simulink model "Green_Ball_Tracking_Mounted"  (R2016a)
settings: configuration reference "AR_Drone_ConfigSet" (kept outside this file)
undefined symbols (not defined in the file): Drone_StateModeType, sigbuilder_block
libraries: simulink x10, AR_Drone_Sensors x2, AR_Drone_Actuators x2, AR_Drone_Video x1, AR_Drone_Positioning x1
(part 1 of 2)
settings Model: DataDictionary=ArDroneDataDictionary.sldd  SimulationMode=external  ExtModeTrigDuration=48000  Creator=nraman  LastModifiedBy=sannem
settings ConfigSetRef: Description='192.168.1.1' 1 17725  DDName=ArDroneDataDictionary.sldd

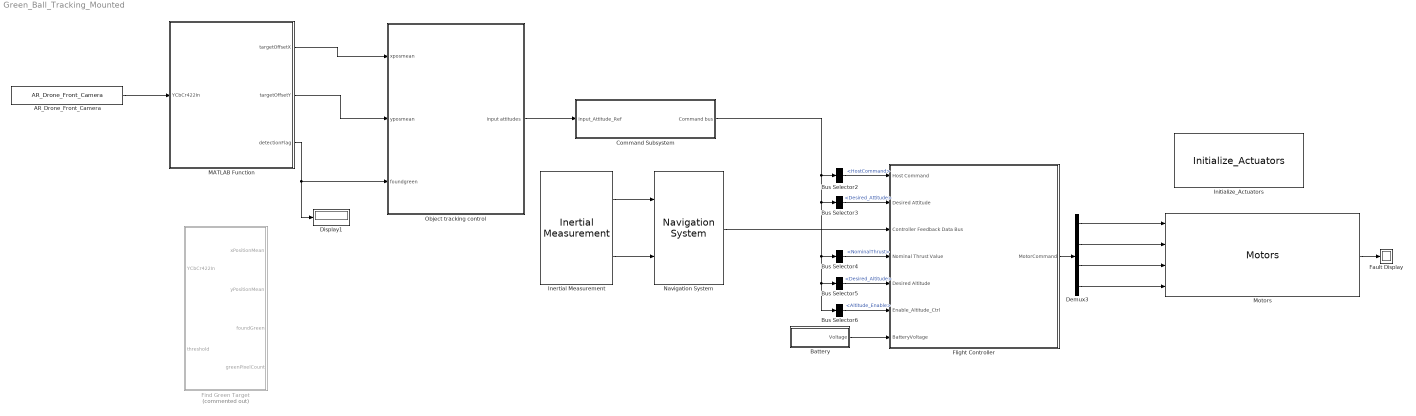
== system Green_Ball_Tracking_Mounted ==
  AR_Drone_Front_Camera : AR_Drone_Video/AR_Drone_Front_Camera  SFunctionSpec=videoGrabImage1(uint8 y1[1843200])  SampleTime=0.1  ShowSpec=off
  Battery : Subsystem
  Bus Selector2 : BusSelector  OutputSignals=HostCommand
  Bus Selector3 : BusSelector  OutputSignals=Desired_Attitude
  Bus Selector4 : BusSelector  OutputSignals=NominalThrust
  Bus Selector5 : BusSelector  OutputSignals=Desired_Altitude
  Bus Selector6 : BusSelector  OutputSignals=Altitude_Enable
  Command Subsystem : Subsystem
  Demux3 : Demux
  Display1 : Display
  Fault Display : Display
  Find Green Target : MATLAB Function  Commented=on  TreatAsAtomicUnit=on  mask(Average Green Position){width=1280, height=720, downScaleFactor=5}
      mask prompts: width "Horizontal resolution"; height "Vertical resolution"; downScaleFactor "Video downscale factor"
      mask help: This block returns the average x and y coordinates of all green pixels within the YCbCr 4:2:2 format input video. Specifying the downscaling factor results in the input video being downsampled by that factor in both horizontal and vertical direction to reduce computation time. The input threshold [0 - 255] controls how "green" high the red and blue shift of the pixels must be before they are no longer considered green.
  Flight Controller : Subsystem
  Inertial Measurement : AR_Drone_Sensors/Inertial Measurement  Ts=1/400
  Initialize_Actuators : AR_Drone_Actuators/Initialize_Actuators  ShowSpec=on
  MATLAB Function : MATLAB Function  TreatAsAtomicUnit=on  mask(AR Drone:  Find Colored Object Position){width=1280, height=720, downScaleFactor=5, cbFloor=0, cbCeiling=117, crFloor=0, crCeiling=117, pixelThreshold=10}
      mask prompts: width "Video input width"; height "Video input height"; downScaleFactor "Video down sample factor"; cbFloor "Blue shift minimum [0-255]"; cbCeiling "Blue shift maximum [0-255]"; crFloor "Red shift minimum [0-255]"; crCeiling "Red shift maximum [0-255]"; pixelThreshold "Minimum object detection pixel count"
      mask help:
      | This MATLAB function block takes an input video stream, down samples in both the horizontal and veritcal direction to reduce the computational demand, and then determines how many pixels fall within the user specified colorspace region and what their average postition is in the video. If you are experiencing some artifacts which are hard to tune out, increase the minimum target pixel count. No target will be registered (detectionFlag = 0) unless as many pixels as you define are found in the target colorspace (detectionFlag = 1).
      | The output x and y position are scaled between -1 and 1.
      |
      | Using the YCbCr colorspace some recommend values are:
      |
      | Green target:
      | cb[min, max] = [0, 100]
      | cr[min, max] = [0, 100]
      |
      | Blue target:
      | cb[min, max] = [155, 255]
      | cr[min, max] = [0, 100]
      |
      | Red target:
      | cb[min, max] = [0, 100]
      | cr[min, max] = [155, 255]
  Motors : AR_Drone_Actuators/Motors
  Navigation System : AR_Drone_Positioning/Navigation System
  Object tracking control : Subsystem  mask{HorRes=1280, VerRes=720}
      mask prompts: HorRes "Horizontal resolution"; VerRes "VerticalResolution"
  wires:
  Motors/1 -> Fault Display/1
  Demux3/1 -> Motors/1
  Demux3/2 -> Motors/2
  Demux3/3 -> Motors/3
  Demux3/4 -> Motors/4
  Inertial Measurement/1 -> Navigation System/1
  Inertial Measurement/2 -> Navigation System/2
  Command Subsystem/1(Command bus) -> Bus Selector2/1, Bus Selector3/1, Bus Selector6/1, Bus Selector5/1, Bus Selector4/1
  Bus Selector4/1 -> Flight Controller/4(Nominal Thrust Value)  "<NominalThrust>"
  Bus Selector5/1 -> Flight Controller/5(Desired Altitude)  "<Desired_Altitude>"
  Bus Selector6/1 -> Flight Controller/6(Enable_Altitude_Ctrl)  "<Altitude_Enable>"
  Flight Controller/1(MotorCommand) -> Demux3/1
  Bus Selector2/1 -> Flight Controller/1(Host Command)  "<HostCommand>"
  Bus Selector3/1 -> Flight Controller/2(Desired Attitude)  "<Desired_Attitude>"
  Navigation System/1 -> Flight Controller/3(Controller Feedback Data Bus)
  AR_Drone_Front_Camera/1 -> MATLAB Function/1(YCbCr422In)
  Object tracking control/1(input attitudes) -> Command Subsystem/1(Input_Attitude_Ref)
  Battery/1(Voltage) -> Flight Controller/7(BatteryVoltage)
  MATLAB Function/1(targetOffsetX) -> Object tracking control/1(xposmean)
  MATLAB Function/2(targetOffsetY) -> Object tracking control/2(yposmean)
  MATLAB Function/3(detectionFlag) -> Display1/1, Object tracking control/3(foundgreen)

== system Green_Ball_Tracking_Mounted/Battery ==
  Battery Voltage Measurement : AR_Drone_Sensors/Battery Voltage Measurement  SFunctionSpec=void BatteryMeasure_step(single y1[1])  SampleTime=-1
  Deci-Volts to Volts : Gain  Gain=1/10
  Display6 : Display
  Voltage : Outport
  wires:
  Deci-Volts to Volts/1 -> Voltage/1, Display6/1
  Battery Voltage Measurement/1 -> Deci-Volts to Volts/1

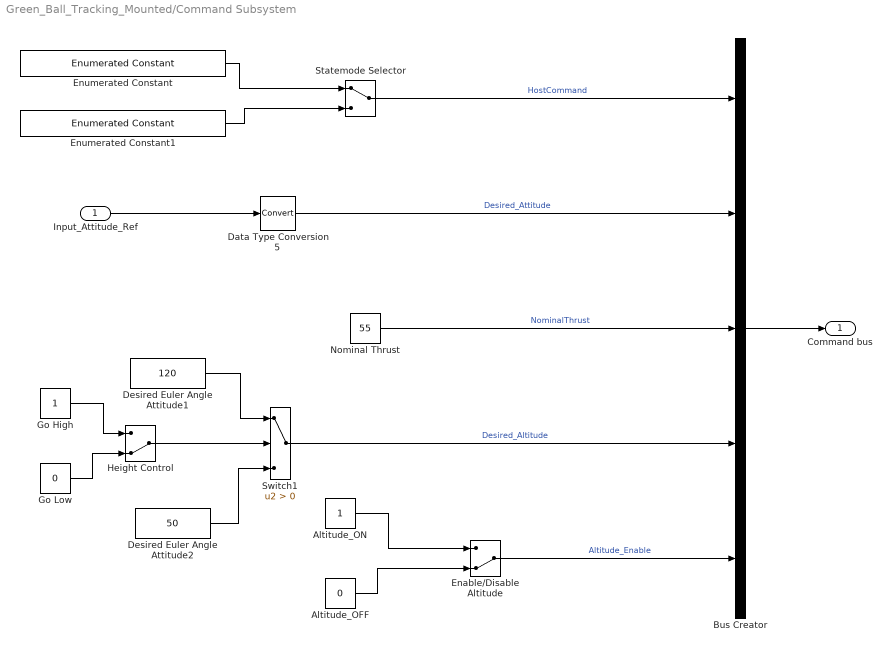
== system Green_Ball_Tracking_Mounted/Command Subsystem ==
  Input_Attitude_Ref : Inport
  Altitude_OFF : Constant  Value=0
  Altitude_ON : Constant
  Bus Creator : BusCreator  Inputs=5
  Data Type Conversion5 : DataTypeConversion
  Desired Euler Angle Attitude1 : Constant  Value=120
  Desired Euler Angle Attitude2 : Constant  Value=50
  Enable/Disable Altitude : ManualSwitch  CurrentSetting=0
  Enumerated Constant : simulink/Sources/Enumerated Constant  OutDataTypeStr=Enum: Drone_StateModeType  Value=Drone_StateModeType.Controlled_Flight  SampleTime=inf
      settings: AttributesFormatString=%<Value>
  Enumerated Constant1 : simulink/Sources/Enumerated Constant  OutDataTypeStr=Enum: Drone_StateModeType  Value=Drone_StateModeType.Landing_Sequence  SampleTime=inf
      settings: AttributesFormatString=%<Value>
  Go High : Constant
  Go Low : Constant  Value=0
  Height Control : ManualSwitch  CurrentSetting=0
  Nominal Thrust : Constant  Value=55
  "Statemode Selector " : ManualSwitch
  Switch1 : Switch  Criteria=u2 > Threshold
  Command bus : Outport
  wires:
  Desired Euler Angle Attitude2/1 -> Switch1/3
  Height Control/1 -> Switch1/2
  Desired Euler Angle Attitude1/1 -> Switch1/1
  Go High/1 -> Height Control/1
  Go Low/1 -> Height Control/2
  Altitude_OFF/1 -> Enable/Disable Altitude/2
  Altitude_ON/1 -> Enable/Disable Altitude/1
  Switch1/1 -> Bus Creator/4  "Desired_Altitude"
  Enable/Disable Altitude/1 -> Bus Creator/5  "Altitude_Enable"
  Nominal Thrust/1 -> Bus Creator/3  "NominalThrust"
  Input_Attitude_Ref/1 -> Data Type Conversion5/1
  Data Type Conversion5/1 -> Bus Creator/2  "Desired_Attitude"
  "Statemode Selector "/1 -> Bus Creator/1  "HostCommand"
  Enumerated Constant/1 -> "Statemode Selector "/1
  Enumerated Constant1/1 -> "Statemode Selector "/2
  Bus Creator/1 -> Command bus/1

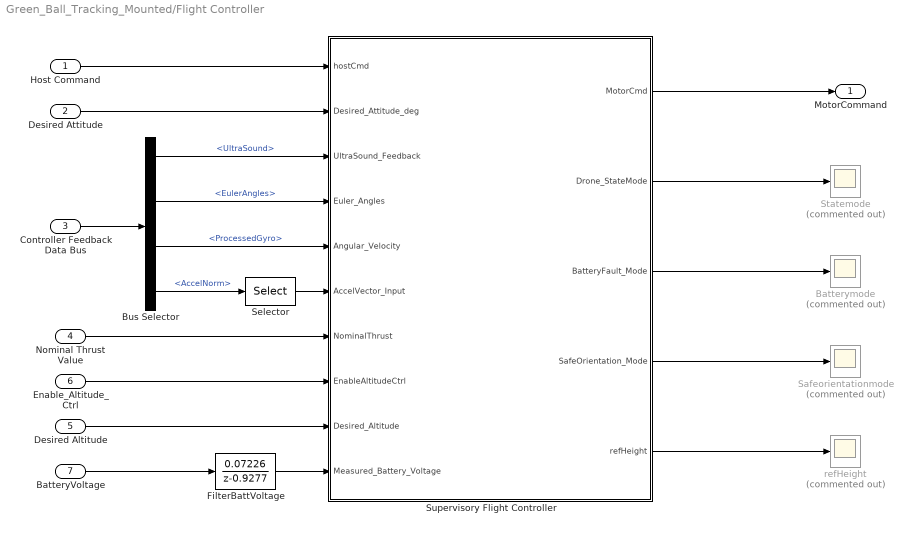
== system Green_Ball_Tracking_Mounted/Flight Controller ==
  Host Command : Inport
  Desired Attitude : Inport  Port=2
  Controller Feedback Data Bus : Inport  Port=3
  Nominal Thrust Value : Inport  Port=4
  Desired Altitude : Inport  Port=5
  Enable_Altitude_Ctrl : Inport  Port=6
  BatteryVoltage : Inport  Port=7
  Batterymode : Scope  Commented=on
  Bus Selector : BusSelector  OutputSignals=UltraSound,EulerAngles,ProcessedGyro,AccelNorm
  FilterBattVoltage : DiscreteTransferFcn  Numerator=[ 0.07226]  Denominator=[1 -0.9277]
  Safeorientationmode : Scope  Commented=on
  Selector : Selector  InputPortWidth=3  IndexOptions=Index vector (dialog)  Indices=[3]  OutputSizes=1
  Statemode : Scope  Commented=on
  Supervisory Flight Controller : Stateflow chart  TreatAsAtomicUnit=on
  refHeight : Scope  Commented=on
  MotorCommand : Outport
  wires:
  Supervisory Flight Controller/1(MotorCmd) -> MotorCommand/1
  Desired Attitude/1 -> Supervisory Flight Controller/2(Desired_Attitude_deg)
  Desired Altitude/1 -> Supervisory Flight Controller/9(Desired_Altitude)
  Supervisory Flight Controller/2(" Drone_StateMode") -> Statemode/1
  Host Command/1 -> Supervisory Flight Controller/1(hostCmd)
  Bus Selector/1 -> Supervisory Flight Controller/3(UltraSound_Feedback)  "<UltraSound>"
  Nominal Thrust Value/1 -> Supervisory Flight Controller/7(NominalThrust)
  Controller Feedback Data Bus/1 -> Bus Selector/1
  Enable_Altitude_Ctrl/1 -> Supervisory Flight Controller/8(EnableAltitudeCtrl)
  BatteryVoltage/1 -> FilterBattVoltage/1
  FilterBattVoltage/1 -> Supervisory Flight Controller/10(Measured_Battery_Voltage)
  Selector/1 -> Supervisory Flight Controller/6(AccelVector_Input)
  Bus Selector/4 -> Selector/1  "<AccelNorm>"
  Bus Selector/2 -> Supervisory Flight Controller/4(Euler_Angles)  "<EulerAngles>"
  Bus Selector/3 -> Supervisory Flight Controller/5(Angular_Velocity)  "<ProcessedGyro>"
  Supervisory Flight Controller/3(" BatteryFault_Mode") -> Batterymode/1
  Supervisory Flight Controller/4(" SafeOrientation_Mode") -> Safeorientationmode/1
  Supervisory Flight Controller/5(refHeight) -> refHeight/1

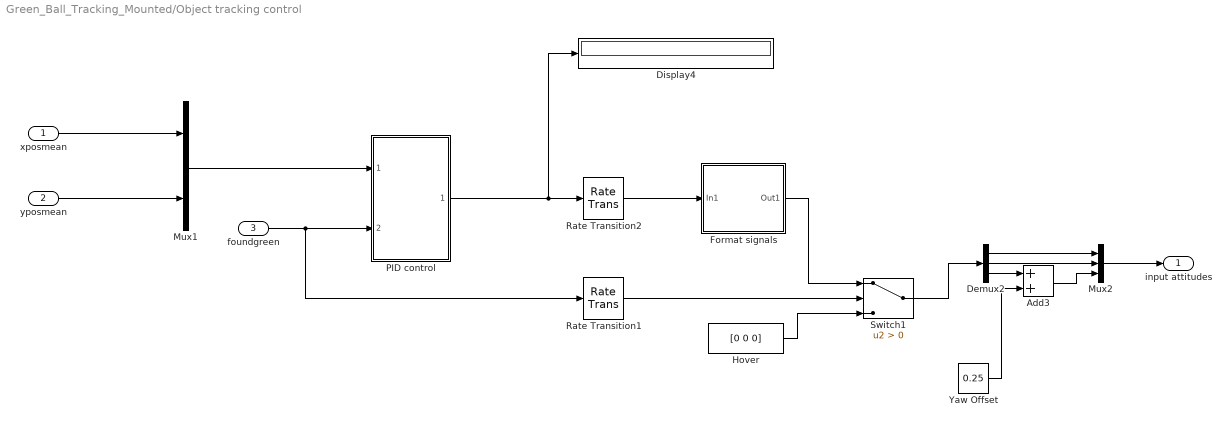
== system Green_Ball_Tracking_Mounted/Object tracking control ==
  xposmean : Inport
  yposmean : Inport  Port=2
  foundgreen : Inport  Port=3
  Add3 : Sum
  Demux2 : Demux  Outputs=3
  Display4 : Display
  Format signals : Subsystem
  Hover : Constant  Value=[0 0 0]
  Mux1 : Mux  Inputs=2
  Mux2 : Mux  Inputs=3
  PID control : Subsystem
  Rate Transition1 : RateTransition
  Rate Transition2 : RateTransition
  Switch1 : Switch  Criteria=u2 > Threshold
  "Yaw Offset " : Constant  Value=0.25
  input attitudes : Outport
  wires:
  Switch1/1 -> Demux2/1
  "Yaw Offset "/1 -> Add3/2
  Demux2/2 -> Mux2/2
  Demux2/1 -> Mux2/1
  Demux2/3 -> Add3/1
  Mux2/1 -> input attitudes/1
  Add3/1 -> Mux2/3
  foundgreen/1 -> PID control/2(Reset Trigger), Rate Transition1/1
  Rate Transition1/1 -> Switch1/2
  Hover/1 -> Switch1/3
  xposmean/1 -> Mux1/1
  yposmean/1 -> Mux1/2
  Rate Transition2/1 -> Format signals/1(In1)
  Format signals/1(Out1) -> Switch1/1
  PID control/1(Control output) -> Display4/1, Rate Transition2/1
  Mux1/1 -> PID control/1(XY Input)

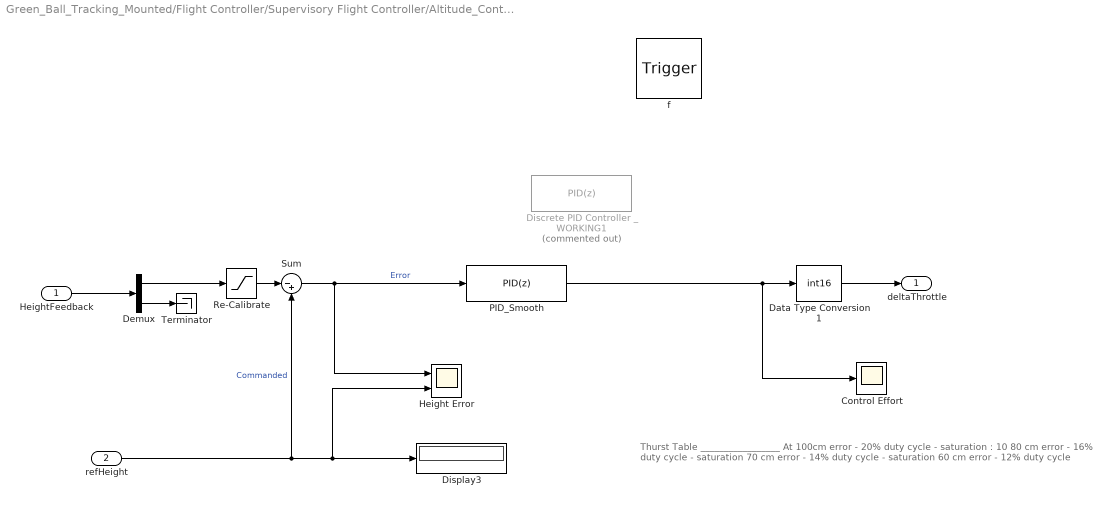
== system Green_Ball_Tracking_Mounted/Flight Controller/Supervisory Flight Controller/Altitude_Control ==
  note: Thurst Table
      | _________________
      | At 100cm error  - 20% duty cycle - saturation : 10
      | 80 cm error - 16% duty cycle - saturation
      | 70 cm error - 14% duty cycle - saturation
      | 60 cm error - 12% duty cycle
  HeightFeedback : Inport  OutDataTypeStr=double  PortDimensions=2
  refHeight : Inport  Port=2  OutDataTypeStr=double  PortDimensions=1
  f : TriggerPort  TriggerType=function-call  VariantControl=Variant
      settings: CopyFcn=Stateflow.SLINSF.SimulinkMan.removeBlockPreDeleteFcn  PreDeleteFcn=Stateflow.SLINSF.SimulinkMan.unsafePredeleteFcn
  Control Effort : Scope
  Data Type Conversion1 : DataTypeConversion  OutDataTypeStr=int16
  Demux : Demux  Outputs=2
  Discrete PID Controller _ WORKING1 : simulink/Continuous/PID Controller  Commented=on  Controller=PID  TimeDomain=Discrete-time  SampleTime=-1  IntegratorMethod=Forward Euler  FilterMethod=Forward Euler  Form=Parallel  UseFilter=on  ControllerParametersSource=internal  P=0.387369235850492*0.7  I=0.018136*4  D=0.819231727791919*0.15  N=12.5907330811849  InitialConditionSource=internal  InitialConditionForIntegrator=0  InitialConditionForFilter=0  ExternalReset=none  LimitOutput=on  UpperSaturationLimit=20  LowerSaturationLimit=-20  LinearizeAsGain=off  AntiWindupMode=clamping  Kb=1  TrackingMode=off  Kt=1  PParamMin=[]  PParamMax=[]  IParamMin=[]  IParamMax=[]  DParamMin=[]  DParamMax=[]  NParamMin=[]  NParamMax=[]  KbParamMin=[]  KbParamMax=[]  KtParamMin=[]  KtParamMax=[]  POutMin=[]  POutMax=[]  IOutMin=[]  IOutMax=[]  DOutMin=[]  DOutMax=[]  NOutMin=[]  NOutMax=[]  KbOutMin=[]  KbOutMax=[]  KtOutMin=[]  KtOutMax=[]  IntegratorOutMin=[]  IntegratorOutMax=[]  FilterOutMin=[]  FilterOutMax=[]  SumOutMin=[]  SumOutMax=[]  SumI1OutMin=[]  SumI1OutMax=[]  SumI2OutMin=[]  SumI2OutMax=[]  SumI3OutMin=[]  SumI3OutMax=[]  SumDOutMin=[]  SumDOutMax=[]  SaturationOutMin=[]  SaturationOutMax=[]  IntegratorContinuousStateAttributes=''  IntegratorStateMustResolveToSignalObject=off  IntegratorRTWStateStorageClass=Auto  FilterContinuousStateAttributes=''  FilterStateMustResolveToSignalObject=off  FilterRTWStateStorageClass=Auto  DifferentiatorICPrevScaledInput=0  DifferentiatorOutMin=[]  DifferentiatorOutMax=[]
  Display3 : Display
  Height Error : Scope  NumInputPorts=2
  PID_Smooth : simulink/Continuous/PID Controller  Controller=PID  TimeDomain=Discrete-time  SampleTime=-1  IntegratorMethod=Forward Euler  FilterMethod=Forward Euler  Form=Parallel  UseFilter=on  ControllerParametersSource=internal  P=0.387369235850492*0.9  I=0.018136*4  D=0.819231727791919*0.2  N=12.5907330811849  InitialConditionSource=internal  InitialConditionForIntegrator=0  InitialConditionForFilter=0  ExternalReset=none  LimitOutput=on  UpperSaturationLimit=20  LowerSaturationLimit=-20  LinearizeAsGain=off  AntiWindupMode=clamping  Kb=1  TrackingMode=off  Kt=1  PParamMin=[]  PParamMax=[]  IParamMin=[]  IParamMax=[]  DParamMin=[]  DParamMax=[]  NParamMin=[]  NParamMax=[]  KbParamMin=[]  KbParamMax=[]  KtParamMin=[]  KtParamMax=[]  POutMin=[]  POutMax=[]  IOutMin=[]  IOutMax=[]  DOutMin=[]  DOutMax=[]  NOutMin=[]  NOutMax=[]  KbOutMin=[]  KbOutMax=[]  KtOutMin=[]  KtOutMax=[]  IntegratorOutMin=[]  IntegratorOutMax=[]  FilterOutMin=[]  FilterOutMax=[]  SumOutMin=[]  SumOutMax=[]  SumI1OutMin=[]  SumI1OutMax=[]  SumI2OutMin=[]  SumI2OutMax=[]  SumI3OutMin=[]  SumI3OutMax=[]  SumDOutMin=[]  SumDOutMax=[]  SaturationOutMin=[]  SaturationOutMax=[]  IntegratorContinuousStateAttributes=''  IntegratorStateMustResolveToSignalObject=off  IntegratorRTWStateStorageClass=Auto  FilterContinuousStateAttributes=''  FilterStateMustResolveToSignalObject=off  FilterRTWStateStorageClass=Auto  DifferentiatorICPrevScaledInput=0  DifferentiatorOutMin=[]  DifferentiatorOutMax=[]
  Re-Calibrate : Saturate  UpperLimit=200  LowerLimit=0  OutMin=0  OutMax=200
      settings: AttributesFormatString=|
      | Upper: %<UpperLimit>
      | Lower %<LowerLimit>
  Sum : Sum  Inputs=|-+
  Terminator : Terminator
  deltaThrottle : Outport  OutDataTypeStr=int16
  wires:
  refHeight/1 -> Sum/2, Height Error/2, Display3/1  "Commanded"
  PID_Smooth/1 -> Control Effort/1, Data Type Conversion1/1
  Data Type Conversion1/1 -> deltaThrottle/1
  HeightFeedback/1 -> Demux/1
  Demux/1 -> Re-Calibrate/1
  Sum/1 -> PID_Smooth/1, Height Error/1  "Error"
  Re-Calibrate/1 -> Sum/1
  Demux/2 -> Terminator/1

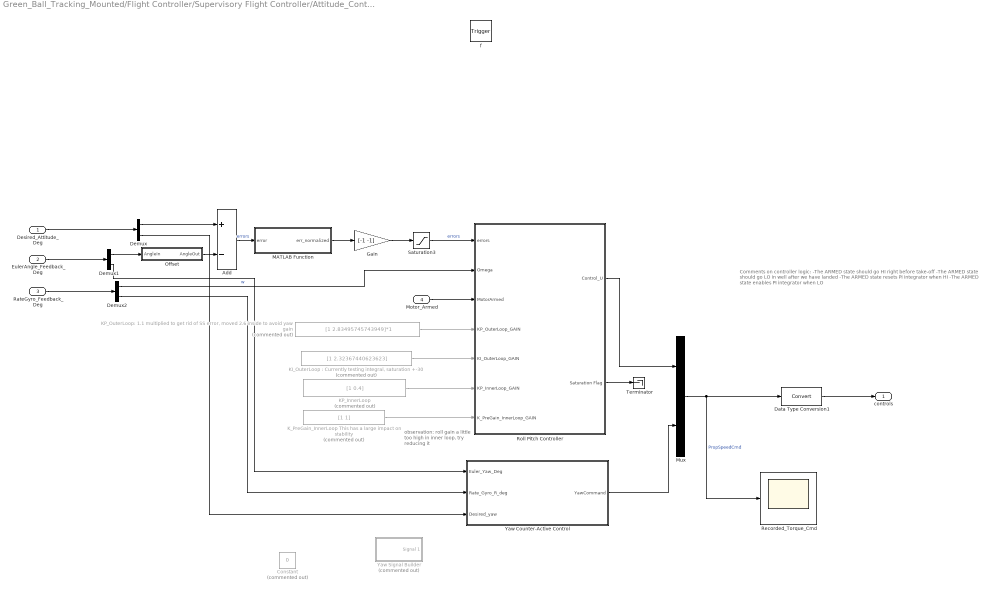
== system Green_Ball_Tracking_Mounted/Flight Controller/Supervisory Flight Controller/Attitude_Control ==
  note: observation:
      | roll gain a little
      | too high in inner
      | loop, try reducing it
  note: Comments on controller logic:
      | -The ARMED state should go HI right before take-off
      | -The  ARMED state should go LO in well after we have landed
      | -The ARMED state resets PI integrator when HI
      | -The ARMED state enables PI integrator when LO
  Desired_Attitude_Deg : Inport  OutDataTypeStr=double  PortDimensions=3
  EulerAngle_Feedback_Deg : Inport  Port=2  OutDataTypeStr=double  PortDimensions=3
  RateGyro_Feedback_Deg : Inport  Port=3  OutDataTypeStr=double  PortDimensions=3
  Motor_Armed : Inport  Port=4  OutDataTypeStr=double  PortDimensions=1
  f : TriggerPort  TriggerType=function-call  VariantControl=Variant
      settings: CopyFcn=Stateflow.SLINSF.SimulinkMan.removeBlockPreDeleteFcn  PreDeleteFcn=Stateflow.SLINSF.SimulinkMan.unsafePredeleteFcn
  Add : Sum  Inputs=+-  AccumDataTypeStr=single  OutDataTypeStr=single
  Constant : Constant  Commented=on  Value=0
  Data Type Conversion1 : DataTypeConversion
  Demux : Demux  Outputs=[2 1]
  Demux1 : Demux  Outputs=[2 1]
  Demux2 : Demux  Outputs=[2 1]
  Gain : Gain  Gain=[-1 -1]
  "KI_OuterLoop : Currently testing integral, saturation +-30" : Constant  Commented=on  Value=[1 2.32367440623623]
  KP_InnerLoop : Constant  Commented=on  Value=[1 0.4]
  "KP_OuterLoop: 1.1 multiplied to get rid of SS error, moved 2.6 inside to avoid yaw gain" : Constant  Commented=on  Value=[1 2.83495745743949]*1
  K_PreGain_InnerLoop This has a large impact on stability : Constant  Commented=on  Value=[1 1]
  MATLAB Function : MATLAB Function  TreatAsAtomicUnit=on
  Mux : Mux  Inputs=2
  Offset : Subsystem
  Recorded_Torque_Cmd : Scope
  Roll Pitch Controller : Subsystem  TreatAsAtomicUnit=on
  Saturation3 : Saturate  UpperLimit=[25 25]  LowerLimit=[-25 -25]  OutDataTypeStr=single
      settings: AttributesFormatString=%<LowerLimit> to %<UpperLimit>
  Terminator : Terminator
  Yaw Counter-Active Control : Subsystem
  "Yaw Signal Builder " : Subsystem  Tag=STV Subsys  Commented=on  LoadFcn=sigbuilder_block('load');  StartFcn=sigbuilder_block('start');  StopFcn=sigbuilder_block('stop');  ClipboardFcn=sigbuilder_block('clipboard');  mask(Sigbuilder block){}
      mask help: Simulink:masks:SigbuilderBlock_MD
      mask init:
      | if ~strcmp(get_param(bdroot(gcbh),'SimulationStatus'),'stopped') tuvar = sigbuilder_block('maskInit'); end
      settings: CopyFcn=sigbuilder_block('copy');  DeleteFcn=sigbuilder_block('delete');  ModelCloseFcn=sigbuilder_block('modelClose');  PreSaveFcn=sigbuilder_block('preSave');  PauseFcn=sigbuilder_block('pause');  ContinueFcn=sigbuilder_block('continue');  NameChangeFcn=sigbuilder_block('namechange');  OpenFcn=sigbuilder_block('open',[437.25 118.5 550.5 394.5 ]);  CloseFcn=sigbuilder_block('close');
      mask Display: plot(0, 0, 100, 100,[2, 2, 32, 32, 2], [68, 8, 8, 68, 68],[32, 2], [38, 38], [32, 19, 2],[53, 60, 44], [32, 17, 17, 2],[16, 16, 31, 31]);txt = getActiveGroup(gcbh);text(2, 100, txt,'verticalAlignment', 'top');
  controls : Outport  OutDataTypeStr=int16  PortDimensions=3  InitialOutput=0
  wires:
  Add/1 -> MATLAB Function/1(error)  "errors"
  Demux1/1 -> Offset/1(AngleIn)
  Demux2/1 -> Roll Pitch Controller/2(Omega)  "w"
  KP_InnerLoop/1 -> Roll Pitch Controller/6(KP_InnerLoop_GAIN)
  "KP_OuterLoop: 1.1 multiplied to get rid of SS error, moved 2.6 inside to avoid yaw gain"/1 -> Roll Pitch Controller/4(KP_OuterLoop_GAIN)
  K_PreGain_InnerLoop This has a large impact on stability/1 -> Roll Pitch Controller/7(K_PreGain_InnerLoop_GAIN)
  "KI_OuterLoop : Currently testing integral, saturation +-30"/1 -> Roll Pitch Controller/5(KI_OuterLoop_GAIN)
  Saturation3/1 -> Roll Pitch Controller/1(errors)  "errors"
  MATLAB Function/1(err_normalized) -> Gain/1
  Gain/1 -> Saturation3/1
  Roll Pitch Controller/2(Saturation Flag) -> Terminator/1
  Demux/1 -> Add/1
  Roll Pitch Controller/1(Control_U) -> Mux/1
  Offset/1(AngleOut) -> Add/2
  Demux2/2 -> Yaw Counter-Active Control/2(Rate_Gyro_R_deg)
  Yaw Counter-Active Control/1(YawCommand) -> Mux/2
  Desired_Attitude_Deg/1 -> Demux/1
  EulerAngle_Feedback_Deg/1 -> Demux1/1
  RateGyro_Feedback_Deg/1 -> Demux2/1
  Motor_Armed/1 -> Roll Pitch Controller/3(MotorArmed)
  Demux1/2 -> Yaw Counter-Active Control/1(Euler_Yaw_Deg)
  Data Type Conversion1/1 -> controls/1
  Mux/1 -> Data Type Conversion1/1, Recorded_Torque_Cmd/1  "PropSpeedCmd"
  Demux/2 -> Yaw Counter-Active Control/3("Desired_yaw ")

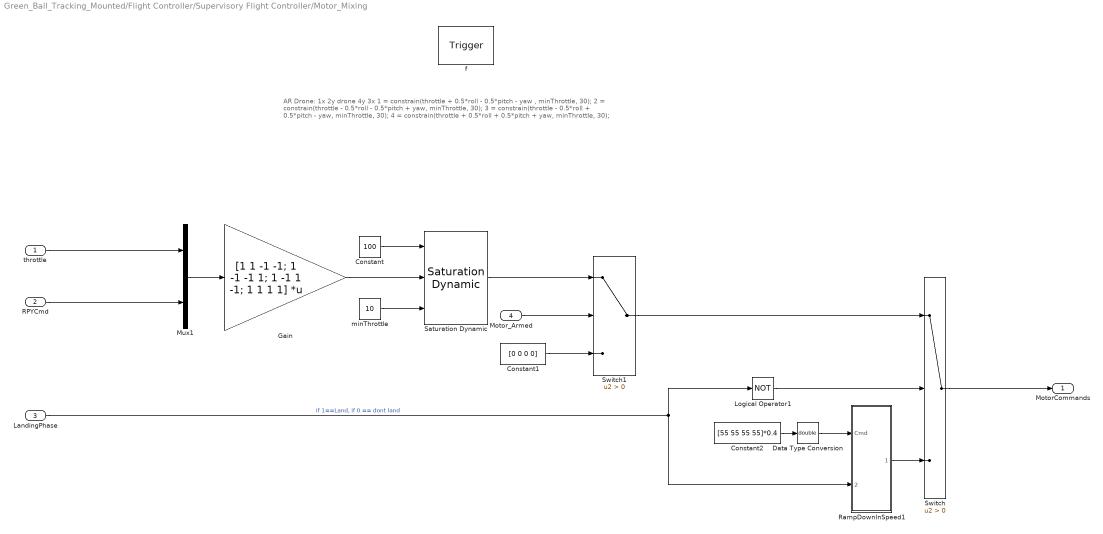
== system Green_Ball_Tracking_Mounted/Flight Controller/Supervisory Flight Controller/Motor_Mixing ==
  note: AR Drone:
      |
      |   1x         2y
      |      drone
      |   4y         3x
      |
      |  1 = constrain(throttle + 0.5*roll - 0.5*pitch - yaw , minThrottle, 30);
      |  2 = constrain(throttle - 0.5*roll - 0.5*pitch + yaw, minThrottle, 30);
      |  3 = constrain(throttle - 0.5*roll + 0.5*pitch - yaw, minThrottle, 30);
      |  4 = constrain(throttle + 0.5*roll + 0.5*pitch + yaw, minThrottle, 30);
  throttle : Inport  OutDataTypeStr=int16  PortDimensions=1
  RPYCmd : Inport  Port=2  OutDataTypeStr=int16  PortDimensions=3
  LandingPhase : Inport  Port=3  OutDataTypeStr=double  PortDimensions=1
  Motor_Armed : Inport  Port=4  OutDataTypeStr=double  PortDimensions=1
  f : TriggerPort  TriggerType=function-call  VariantControl=Variant
      settings: CopyFcn=Stateflow.SLINSF.SimulinkMan.removeBlockPreDeleteFcn  PreDeleteFcn=Stateflow.SLINSF.SimulinkMan.unsafePredeleteFcn
  Constant : Constant  Value=100  OutDataTypeStr=int16  SampleTime=-1
  Constant1 : Constant  Value=[0 0 0 0]  OutDataTypeStr=int16
  Constant2 : Constant  Value=[55 55 55 55]*0.4
  Data Type Conversion : DataTypeConversion  OutDataTypeStr=double
  Gain : Gain  Gain=[1 1 -1 -1; 1 -1 -1 1; 1 -1 1 -1; 1 1 1 1]  Multiplication=Matrix(K*u)  ParamDataTypeStr=int16  OutDataTypeStr=int16
  Logical Operator1 : Logic  Operator=NOT  AllPortsSameDT=off  OutDataTypeStr=boolean
  Mux1 : Mux  Inputs=2
  RampDownInSpeed1 : MATLAB Function  TreatAsAtomicUnit=on
  Saturation Dynamic : simulink/Discontinuities/Saturation Dynamic  OutMin=[]  OutMax=[]  OutDataTypeStr=Inherit: Same as second input  OutDataType=fixdt(1, 16)  OutScaling=2^-10  DoSatur=off
  Switch : Switch  Criteria=u2 > Threshold
  Switch1 : Switch  Criteria=u2 > Threshold
  minThrottle : Constant  Value=10  OutDataTypeStr=int16
  MotorCommands : Outport  InitialOutput=0
  wires:
  RPYCmd/1 -> Mux1/2
  minThrottle/1 -> Saturation Dynamic/3
  Constant/1 -> Saturation Dynamic/1
  Mux1/1 -> Gain/1
  Gain/1 -> Saturation Dynamic/2
  throttle/1 -> Mux1/1
  Data Type Conversion/1 -> RampDownInSpeed1/1(Cmd)
  RampDownInSpeed1/1(motorCmd) -> Switch/3
  Constant2/1 -> Data Type Conversion/1
  LandingPhase/1 -> RampDownInSpeed1/2(stopCmd), Logical Operator1/1  "if 1==Land, if 0 == dont land"
  Switch/1 -> MotorCommands/1
  Logical Operator1/1 -> Switch/2
  Saturation Dynamic/1 -> Switch1/1
  Motor_Armed/1 -> Switch1/2
  Constant1/1 -> Switch1/3
  Switch1/1 -> Switch/1

== system Green_Ball_Tracking_Mounted/Object tracking control/Format signals ==
  In1 : Inport
  Constant : Constant  Value=0
  Demux : Demux  Outputs=2
  Mux : Mux  Inputs=3
  Out1 : Outport
  wires:
  Demux/2 -> Mux/2
  Mux/1 -> Out1/1
  Constant/1 -> Mux/1
  Demux/1 -> Mux/3
  In1/1 -> Demux/1

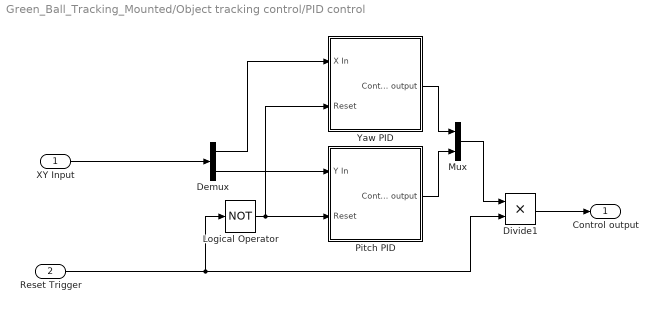
== system Green_Ball_Tracking_Mounted/Object tracking control/PID control ==
  XY Input : Inport
  Reset Trigger : Inport  Port=2
  Demux : Demux  Outputs=2
  Divide1 : Product  Inputs=**
  Logical Operator : Logic  Operator=NOT  Inputs=1  AllPortsSameDT=off  OutDataTypeStr=boolean
  Mux : Mux  Inputs=2
  Pitch PID : Subsystem  mask(PID controller){P=0, I=20, D=0, N=100}
      mask prompts: P "Proportional gain"; I "Integral gain"; D "Derivative gain"; N "Filer coefficient"
      mask help: This is the PID controller used for tracking the target, use the parameter values below to tune the PID in real time.
  Yaw PID : Subsystem  mask(PID controller){P=-3, I=0, D=0, N=100}
      mask prompts: P "Proportional gain"; I "Integral gain"; D "Derivative gain"; N "Filer coefficient"
      mask help: This is the PID controller used for tracking the target, use the parameter values below to tune the PID in real time.
  Control output : Outport
  wires:
  Pitch PID/1(Control output) -> Mux/2
  Yaw PID/1(Control output) -> Mux/1
  Demux/2 -> Pitch PID/1(Y In)
  Demux/1 -> Yaw PID/1(X In)
  Divide1/1 -> Control output/1
  Reset Trigger/1 -> Divide1/2, Logical Operator/1
  Logical Operator/1 -> Yaw PID/2(Reset), Pitch PID/2(Reset)
  Mux/1 -> Divide1/1
  XY Input/1 -> Demux/1

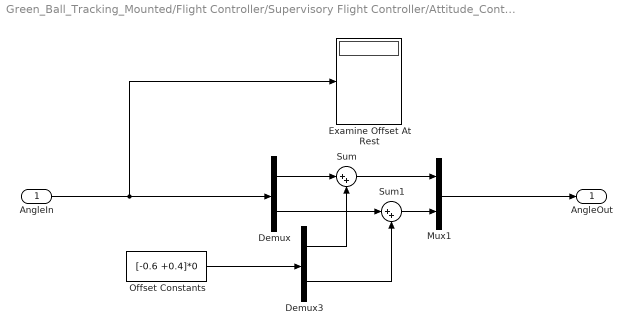
== system Green_Ball_Tracking_Mounted/Flight Controller/Supervisory Flight Controller/Attitude_Control/Offset ==
  AngleIn : Inport
  Demux : Demux  Outputs=2
  Demux3 : Demux  Outputs=2
  Examine Offset At Rest : Display
  Mux1 : Mux  Inputs=2
  Offset Constants : Constant  Value=[-0.6 +0.4]*0  OutDataTypeStr=single
  Sum : Sum  Inputs=|++
  Sum1 : Sum  Inputs=|++
  AngleOut : Outport
  wires:
  Mux1/1 -> AngleOut/1
  Sum/1 -> Mux1/1
  Sum1/1 -> Mux1/2
  Demux/2 -> Sum1/1
  AngleIn/1 -> Examine Offset At Rest/1, Demux/1
  Demux3/2 -> Sum1/2
  Demux3/1 -> Sum/2
  Demux/1 -> Sum/1
  Offset Constants/1 -> Demux3/1

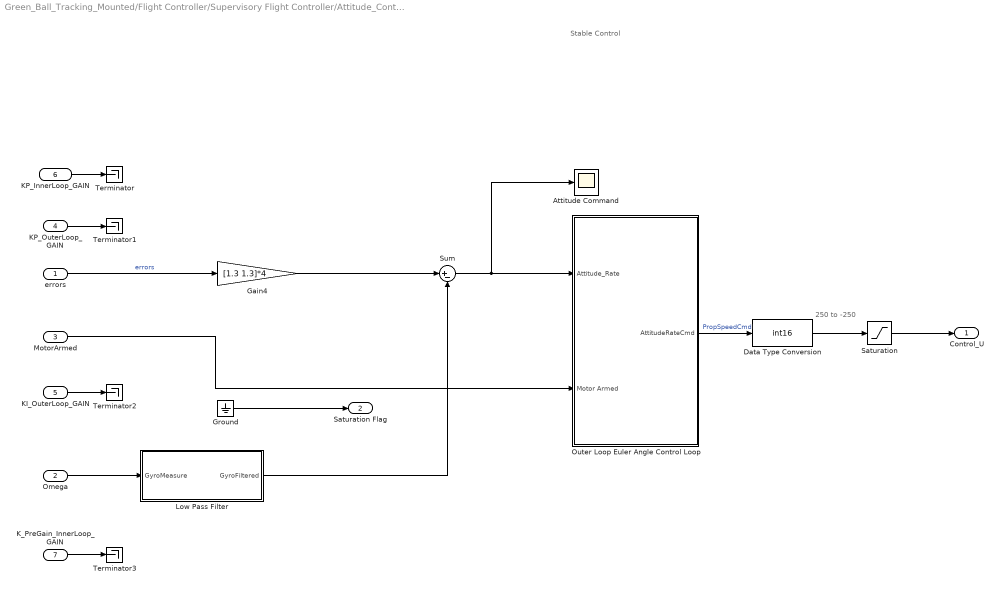
== system Green_Ball_Tracking_Mounted/Flight Controller/Supervisory Flight Controller/Attitude_Control/Roll Pitch Controller ==
  note: 250 to -250
  note: Stable Control
  errors : Inport
  Omega : Inport  Port=2
  MotorArmed : Inport  Port=3
  KP_OuterLoop_GAIN : Inport  Port=4
  KI_OuterLoop_GAIN : Inport  Port=5
  KP_InnerLoop_GAIN : Inport  Port=6
  K_PreGain_InnerLoop_GAIN : Inport  Port=7
  Attitude Command : Scope
  Data Type Conversion : DataTypeConversion  OutDataTypeStr=int16  RndMeth=Nearest
  Gain4 : Gain  Gain=[1.3 1.3]*4
  Ground : Ground
  Low Pass Filter : Subsystem
  Outer Loop Euler Angle Control Loop : Subsystem
  Saturation : Saturate  UpperLimit=250  LowerLimit=-250  OutDataTypeStr=int16
      settings: AttributesFormatString=%<LowerLimit>\nto\n%<UpperLimit>
  Sum : Sum  Inputs=|+-
  Terminator{,1..3} (4 alike) : Terminator
  Control_U : Outport
  Saturation Flag : Outport  Port=2
  wires:
  Saturation/1 -> Control_U/1
  Data Type Conversion/1 -> Saturation/1
  Outer Loop Euler Angle Control Loop/1(AttitudeRateCmd) -> Data Type Conversion/1  "PropSpeedCmd"
  MotorArmed/1 -> Outer Loop Euler Angle Control Loop/2(Motor Armed)
  Ground/1 -> Saturation Flag/1
  Omega/1 -> Low Pass Filter/1(GyroMeasure)
  errors/1 -> Gain4/1  "errors"
  Sum/1 -> Attitude Command/1, Outer Loop Euler Angle Control Loop/1(Attitude_Rate)
  Gain4/1 -> Sum/1
  Low Pass Filter/1(GyroFiltered) -> Sum/2
  KP_InnerLoop_GAIN/1 -> Terminator/1
  KP_OuterLoop_GAIN/1 -> Terminator1/1
  KI_OuterLoop_GAIN/1 -> Terminator2/1
  K_PreGain_InnerLoop_GAIN/1 -> Terminator3/1

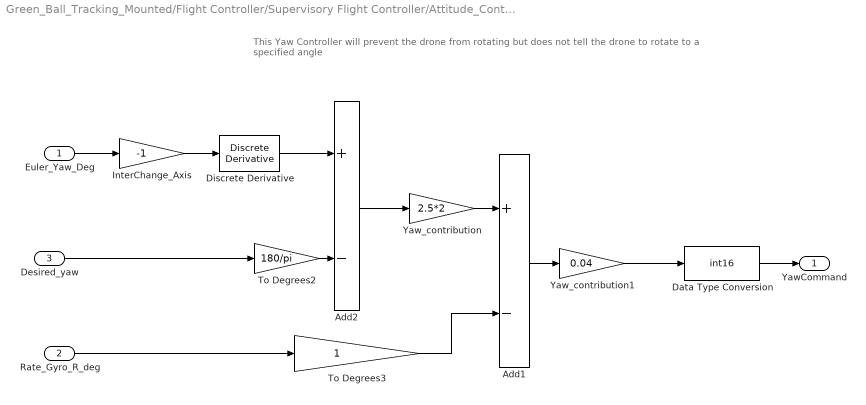
== system Green_Ball_Tracking_Mounted/Flight Controller/Supervisory Flight Controller/Attitude_Control/Yaw Counter-Active Control ==
  note: This Yaw Controller will prevent the drone from
      | rotating but does not tell the drone to rotate to a specified angle
  Euler_Yaw_Deg : Inport
  Rate_Gyro_R_deg : Inport  Port=2
  "Desired_yaw " : Inport  Port=3
  Add1 : Sum  Inputs=+-  AccumDataTypeStr=single  OutDataTypeStr=single
  Add2 : Sum  Inputs=+-  AccumDataTypeStr=single  OutDataTypeStr=single
  Data Type Conversion : DataTypeConversion  OutDataTypeStr=int16
  Discrete Derivative : simulink/Discrete/Discrete Derivative  gainval=1.0  ICPrevScaledInput=0.0  InputProcessing=Inherited  OutMin=[]  OutMax=[]  OutDataType=fixdt(1, 16)  OutScaling=2^-10  DoSatur=off
  InterChange_Axis : Gain  Gain=-1  ParamDataTypeStr=single  OutDataTypeStr=single
      settings: AttributesFormatString=%<Gain>
  To Degrees2 : Gain  Gain=180/pi  ParamDataTypeStr=single  OutDataTypeStr=single
      settings: AttributesFormatString=%<Gain>
  To Degrees3 : Gain  ParamDataTypeStr=single  OutDataTypeStr=single
      settings: AttributesFormatString=%<Gain>
  Yaw_contribution : Gain  Gain=2.5*2  ParamDataTypeStr=single  OutDataTypeStr=single
      settings: AttributesFormatString=%<Gain>
  Yaw_contribution1 : Gain  Gain=0.04  ParamDataTypeStr=single  OutDataTypeStr=single
      settings: AttributesFormatString=%<Gain>
  YawCommand : Outport
  wires:
  Yaw_contribution1/1 -> Data Type Conversion/1
  To Degrees3/1 -> Add1/2
  Euler_Yaw_Deg/1 -> InterChange_Axis/1
  Add1/1 -> Yaw_contribution1/1
  Yaw_contribution/1 -> Add1/1
  Add2/1 -> Yaw_contribution/1
  InterChange_Axis/1 -> Discrete Derivative/1
  Discrete Derivative/1 -> Add2/1
  To Degrees2/1 -> Add2/2
  "Desired_yaw "/1 -> To Degrees2/1
  Rate_Gyro_R_deg/1 -> To Degrees3/1
  Data Type Conversion/1 -> YawCommand/1

== system Green_Ball_Tracking_Mounted/Flight Controller/Supervisory Flight Controller/Attitude_Control/Yaw Signal Builder  ==
  Demux : Demux  Tag=STV Demux  Outputs=1
  FromWs : FromWorkspace  Tag=STV FromWs  VariableName=tuvar
      SigBuilderData=|
      | common.afterFinalStr = 'Extrapolate'
      | common.sampleTime = '-1'
      | dataSet.timeRange = [0 20]
      | dataSet.name = 'Group 1'
      | sbobj.Groups.Name = 'Group 1'
      | sbobj.Groups.Signals.Name = 'Signal 1'
      | sbobj.Groups.Signals.XData = [0 10 10 12.5 12.5 15 15 20]
      | sbobj.Groups.Signals.YData = [0 0 2 2 -2 -2 0 0]
      | sbobj.Groups.TimeRange = [0 20]
  Signal 1 : Outport  Tag=STV Outport
  wires:
  Demux/1 -> Signal 1/1
  FromWs/1 -> Demux/1

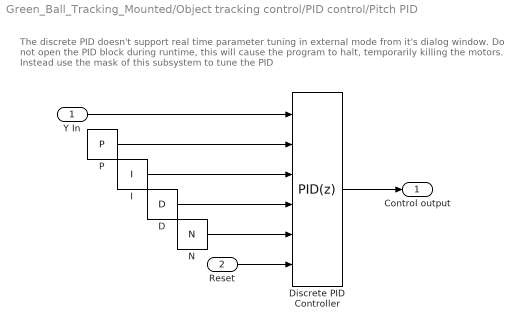
== system Green_Ball_Tracking_Mounted/Object tracking control/PID control/Pitch PID ==
  note: The discrete PID doesn't support real time parameter tuning in external mode from it's dialog window.
      | Do not open the PID block during runtime, this will cause the program to halt, temporarily killing the motors.
      | Instead use the mask of this subsystem to tune the PID
  Y In : Inport
  Reset : Inport  Port=2
  D : Constant  Value=D
  Discrete PID Controller : simulink/Continuous/PID Controller  Controller=PID  TimeDomain=Discrete-time  SampleTime=-1  IntegratorMethod=Forward Euler  FilterMethod=Forward Euler  Form=Parallel  UseFilter=on  ControllerParametersSource=external  P=1  I=1  D=0  N=100  InitialConditionSource=internal  InitialConditionForIntegrator=0  InitialConditionForFilter=0  ExternalReset=level  LimitOutput=off  UpperSaturationLimit=inf  LowerSaturationLimit=-inf  LinearizeAsGain=off  AntiWindupMode=none  Kb=1  TrackingMode=off  Kt=1  PParamMin=[]  PParamMax=[]  IParamMin=[]  IParamMax=[]  DParamMin=[]  DParamMax=[]  NParamMin=[]  NParamMax=[]  KbParamMin=[]  KbParamMax=[]  KtParamMin=[]  KtParamMax=[]  POutMin=[]  POutMax=[]  IOutMin=[]  IOutMax=[]  DOutMin=[]  DOutMax=[]  NOutMin=[]  NOutMax=[]  KbOutMin=[]  KbOutMax=[]  KtOutMin=[]  KtOutMax=[]  IntegratorOutMin=[]  IntegratorOutMax=[]  FilterOutMin=[]  FilterOutMax=[]  SumOutMin=[]  SumOutMax=[]  SumI1OutMin=[]  SumI1OutMax=[]  SumI2OutMin=[]  SumI2OutMax=[]  SumI3OutMin=[]  SumI3OutMax=[]  SumDOutMin=[]  SumDOutMax=[]  SaturationOutMin=[]  SaturationOutMax=[]  IntegratorContinuousStateAttributes=''  IntegratorStateMustResolveToSignalObject=off  IntegratorRTWStateStorageClass=Auto  FilterContinuousStateAttributes=''  FilterStateMustResolveToSignalObject=off  FilterRTWStateStorageClass=Auto  DifferentiatorICPrevScaledInput=0  DifferentiatorOutMin=[]  DifferentiatorOutMax=[]
  I : Constant  Value=I
  N : Constant  Value=N
  "P " : Constant  Value=P
  Control output : Outport
  wires:
  Discrete PID Controller/1 -> Control output/1
  Reset/1 -> Discrete PID Controller/6
  Y In/1 -> Discrete PID Controller/1
  I/1 -> Discrete PID Controller/3
  D/1 -> Discrete PID Controller/4
  N/1 -> Discrete PID Controller/5
  "P "/1 -> Discrete PID Controller/2

== system Green_Ball_Tracking_Mounted/Object tracking control/PID control/Yaw PID ==
  note: The discrete PID doesn't support real time parameter tuning in external mode from it's dialog window.
      | Do not open the PID block during runtime, this will cause the program to halt, temporarily killing the motors.
      | Instead use the mask of this subsystem to tune the PID
  X In : Inport
  Reset : Inport  Port=2
  D : Constant  Value=D
  Discrete PID Controller : simulink/Continuous/PID Controller  Controller=PID  TimeDomain=Discrete-time  SampleTime=-1  IntegratorMethod=Forward Euler  FilterMethod=Forward Euler  Form=Parallel  UseFilter=on  ControllerParametersSource=external  P=1  I=1  D=0  N=100  InitialConditionSource=internal  InitialConditionForIntegrator=0  InitialConditionForFilter=0  ExternalReset=level  LimitOutput=off  UpperSaturationLimit=inf  LowerSaturationLimit=-inf  LinearizeAsGain=off  AntiWindupMode=none  Kb=1  TrackingMode=off  Kt=1  PParamMin=[]  PParamMax=[]  IParamMin=[]  IParamMax=[]  DParamMin=[]  DParamMax=[]  NParamMin=[]  NParamMax=[]  KbParamMin=[]  KbParamMax=[]  KtParamMin=[]  KtParamMax=[]  POutMin=[]  POutMax=[]  IOutMin=[]  IOutMax=[]  DOutMin=[]  DOutMax=[]  NOutMin=[]  NOutMax=[]  KbOutMin=[]  KbOutMax=[]  KtOutMin=[]  KtOutMax=[]  IntegratorOutMin=[]  IntegratorOutMax=[]  FilterOutMin=[]  FilterOutMax=[]  SumOutMin=[]  SumOutMax=[]  SumI1OutMin=[]  SumI1OutMax=[]  SumI2OutMin=[]  SumI2OutMax=[]  SumI3OutMin=[]  SumI3OutMax=[]  SumDOutMin=[]  SumDOutMax=[]  SaturationOutMin=[]  SaturationOutMax=[]  IntegratorContinuousStateAttributes=''  IntegratorStateMustResolveToSignalObject=off  IntegratorRTWStateStorageClass=Auto  FilterContinuousStateAttributes=''  FilterStateMustResolveToSignalObject=off  FilterRTWStateStorageClass=Auto  DifferentiatorICPrevScaledInput=0  DifferentiatorOutMin=[]  DifferentiatorOutMax=[]
  I : Constant  Value=I
  N : Constant  Value=N
  "P " : Constant  Value=P
  Control output : Outport
  wires:
  Discrete PID Controller/1 -> Control output/1
  Reset/1 -> Discrete PID Controller/6
  X In/1 -> Discrete PID Controller/1
  I/1 -> Discrete PID Controller/3
  D/1 -> Discrete PID Controller/4
  N/1 -> Discrete PID Controller/5
  "P "/1 -> Discrete PID Controller/2

== system Green_Ball_Tracking_Mounted/Flight Controller/Supervisory Flight Controller/Attitude_Control/Roll Pitch Controller/Low Pass Filter ==
  GyroMeasure : Inport
  Demux : Demux  Outputs=2
  Digital Low Pass Filter1 : DiscreteTransferFcn  Numerator=[0.04877]  Denominator=[1 -0.9512]  OutDataTypeStr=int16
  Digital Low Pass Filter2 : DiscreteTransferFcn  Numerator=[0.04877]  Denominator=[1 -0.9512]  OutDataTypeStr=int16
  Digital Low Pass Filter3 : DiscreteTransferFcn  Commented=on  Numerator=[0.04877]  Denominator=[1 -0.9512]  OutDataTypeStr=int16
  Mux3 : Mux  Inputs=2
  GyroFiltered : Outport
  wires:
  Mux3/1 -> GyroFiltered/1
  Demux/1 -> Digital Low Pass Filter2/1
  GyroMeasure/1 -> Demux/1
  Demux/2 -> Digital Low Pass Filter1/1
  Digital Low Pass Filter2/1 -> Mux3/1
  Digital Low Pass Filter1/1 -> Mux3/2

== system Green_Ball_Tracking_Mounted/Flight Controller/Supervisory Flight Controller/Attitude_Control/Roll Pitch Controller/Outer Loop Euler Angle Control Loop ==
  Attitude_Rate : Inport
  Motor Armed : Inport  Port=2
  Logical Operator : Logic  Operator=NOT  AllPortsSameDT=off  OutDataTypeStr=boolean
  PID Controller : simulink/Continuous/PID Controller  Commented=on  Controller=PID  TimeDomain=Discrete-time  SampleTime=-1  IntegratorMethod=Forward Euler  FilterMethod=Forward Euler  Form=Parallel  UseFilter=on  ControllerParametersSource=internal  P=2.8281  I=28.23  D=0.023379  N=0.0076593  InitialConditionSource=internal  InitialConditionForIntegrator=0  InitialConditionForFilter=0  ExternalReset=level  LimitOutput=on  UpperSaturationLimit=30  LowerSaturationLimit=-30  LinearizeAsGain=on  AntiWindupMode=clamping  Kb=1  TrackingMode=off  Kt=1  PParamMin=[]  PParamMax=[]  IParamMin=[]  IParamMax=[]  DParamMin=[]  DParamMax=[]  NParamMin=[]  NParamMax=[]  KbParamMin=[]  KbParamMax=[]  KtParamMin=[]  KtParamMax=[]  POutMin=[]  POutMax=[]  IOutMin=[]  IOutMax=[]  DOutMin=[]  DOutMax=[]  NOutMin=[]  NOutMax=[]  KbOutMin=[]  KbOutMax=[]  KtOutMin=[]  KtOutMax=[]  IntegratorOutMin=[]  IntegratorOutMax=[]  FilterOutMin=[]  FilterOutMax=[]  SumOutMin=[]  SumOutMax=[]  SumI1OutMin=[]  SumI1OutMax=[]  SumI2OutMin=[]  SumI2OutMax=[]  SumI3OutMin=[]  SumI3OutMax=[]  SumDOutMin=[]  SumDOutMax=[]  SaturationOutMin=[]  SaturationOutMax=[]  IntegratorContinuousStateAttributes=''  IntegratorStateMustResolveToSignalObject=off  IntegratorRTWStateStorageClass=Auto  FilterContinuousStateAttributes=''  FilterStateMustResolveToSignalObject=off  FilterRTWStateStorageClass=Auto  DifferentiatorICPrevScaledInput=0  DifferentiatorOutMin=[]  DifferentiatorOutMax=[]
  PID Controller1 : simulink/Continuous/PID Controller  Controller=PID  TimeDomain=Discrete-time  SampleTime=-1  IntegratorMethod=Forward Euler  FilterMethod=Forward Euler  Form=Parallel  UseFilter=on  ControllerParametersSource=internal  P=0.10084*2  I=0.13631*2  D=-0.011755  N=5  InitialConditionSource=internal  InitialConditionForIntegrator=0  InitialConditionForFilter=0  ExternalReset=level  LimitOutput=on  UpperSaturationLimit=30  LowerSaturationLimit=-30  LinearizeAsGain=on  AntiWindupMode=clamping  Kb=1  TrackingMode=off  Kt=1  PParamMin=[]  PParamMax=[]  IParamMin=[]  IParamMax=[]  DParamMin=[]  DParamMax=[]  NParamMin=[]  NParamMax=[]  KbParamMin=[]  KbParamMax=[]  KtParamMin=[]  KtParamMax=[]  POutMin=[]  POutMax=[]  IOutMin=[]  IOutMax=[]  DOutMin=[]  DOutMax=[]  NOutMin=[]  NOutMax=[]  KbOutMin=[]  KbOutMax=[]  KtOutMin=[]  KtOutMax=[]  IntegratorOutMin=[]  IntegratorOutMax=[]  FilterOutMin=[]  FilterOutMax=[]  SumOutMin=[]  SumOutMax=[]  SumI1OutMin=[]  SumI1OutMax=[]  SumI2OutMin=[]  SumI2OutMax=[]  SumI3OutMin=[]  SumI3OutMax=[]  SumDOutMin=[]  SumDOutMax=[]  SaturationOutMin=[]  SaturationOutMax=[]  IntegratorContinuousStateAttributes=''  IntegratorStateMustResolveToSignalObject=off  IntegratorRTWStateStorageClass=Auto  FilterContinuousStateAttributes=''  FilterStateMustResolveToSignalObject=off  FilterRTWStateStorageClass=Auto  DifferentiatorICPrevScaledInput=0  DifferentiatorOutMin=[]  DifferentiatorOutMax=[]
  AttitudeRateCmd : Outport
  wires:
  PID Controller1/1 -> AttitudeRateCmd/1  "AttitudeRateCmd"
  Motor Armed/1 -> Logical Operator/1
  Logical Operator/1 -> PID Controller1/2
  Attitude_Rate/1 -> PID Controller1/1

== matlab function Green_Ball_Tracking_Mounted/Find Green Target ==
  data: YCbCr422In input; xPositionMean output; threshold input; yPositionMean output; foundGreen output; greenPixelCount output; width parameter; height parameter; downScaleFactor parameter
function [xPositionMean, yPositionMean, foundGreen,greenPixelCount] = AverageGreenPosition2(YCbCr422In,threshold,width, height, downScaleFactor)

xPosition = 0;
yPosition = 0;
xPositionMean = -1;
yPositionMean = -1;
greenPixelCount = 0;
foundGreen = 0;

for verticalIndex = 1 : 1 : height/downScaleFactor;             % indexing for downsampled vertical direction
    for horizontalIndex = 1 : 1 : (width / 2)/downScaleFactor;  % indexing for downsampled horizontal direction
        index = 4 * (downScaleFactor * (verticalIndex - 1) * (width / 2) + downScaleFactor * horizontalIndex) - 3;  % translate the horizontal and vertical indexes into the index into the video input
        pixel = double([YCbCr422In(index) YCbCr422In(index+1) YCbCr422In(index+2) YCbCr422In(index+3)]);    % retrieve the pixel data and convert for calculation

        if ( pixel(1)  <= threshold && pixel (3) <= threshold )

            greenPixelCount = greenPixelCount + 1;
            xPosition = xPosition + horizontalIndex * downScaleFactor;
            yPosition = yPosition + verticalIndex * downScaleFactor;
        end
    end
end
% compute the average green pixel position
if greenPixelCount > 0
    xPositionMean = 2 * xPosition / greenPixelCount;     %convert back to full width resolution
    yPositionMean = yPosition / greenPixelCount;
    foundGreen = 1;
end
end

== matlab function Green_Ball_Tracking_Mounted/MATLAB Function ==
  data: YCbCr422In input; targetOffsetX output; targetOffsetY output; detectionFlag output; cbFloor parameter; cbCeiling parameter; crFloor parameter; crCeiling parameter; downScaleFactor parameter; height parameter; width parameter; pixelThreshold parameter
function [targetOffsetX, targetOffsetY, detectionFlag]  = coloredObjectPosition(YCbCr422In,cbFloor, cbCeiling, crFloor, crCeiling, downScaleFactor, height, width, pixelThreshold)

xPositionSum = 0;
yPositionSum = 0;
targetOffsetX = 0;
targetOffsetY = 0;
targetPixelCount = 0;
detectionFlag = 0;

for verticalIndex = 1 : 1 : height/downScaleFactor;             % indexing for downsampled vertical direction
    for horizontalIndex = 1 : 1 : (width / 2)/downScaleFactor;  % indexing for downsampled horizontal direction
        index = 4 * (downScaleFactor * (verticalIndex - 1) * (width / 2) + downScaleFactor * horizontalIndex) - 3;  % translate the horizontal and vertical indexes into the index into the video input
        pixel = double([YCbCr422In(index) YCbCr422In(index+1) YCbCr422In(index+2) YCbCr422In(index+3)]);    % retrieve the pixel data and convert for calculation

        %% verify whether this pixel is within the user specified region of the YCbCr colorspace
        if ( pixel(1)  >= cbFloor && pixel(1)  <= cbCeiling && ...
             pixel(3)  >= crFloor && pixel(3)  <= crCeiling  )

            targetPixelCount = targetPixelCount + 1;
            xPositionSum = xPositionSum + 2 * horizontalIndex * downScaleFactor;
            yPositionSum = yPositionSum + verticalIndex * downScaleFactor;
        end
    end
end

% compute the average green pixel position
if targetPixelCount > pixelThreshold
    detectionFlag = 1;
    targetOffsetX = xPositionSum / targetPixelCount / (0.5 * width) - 1;     
    targetOffsetY = -(yPositionSum / targetPixelCount / (0.5 * height) - 1);
else
    % not enough pixels were target pixels:

end

end
